simulink model "Model_2b_H2_batteries_secundary_clean"  (R2019a)
settings: Solver=FixedStepAuto  StartTime=0.0  StopTime=8760  FixedStep=1  RelTol=1e-3
libraries: simulink x8
settings Model: Creator=senja  LastModifiedBy=senja

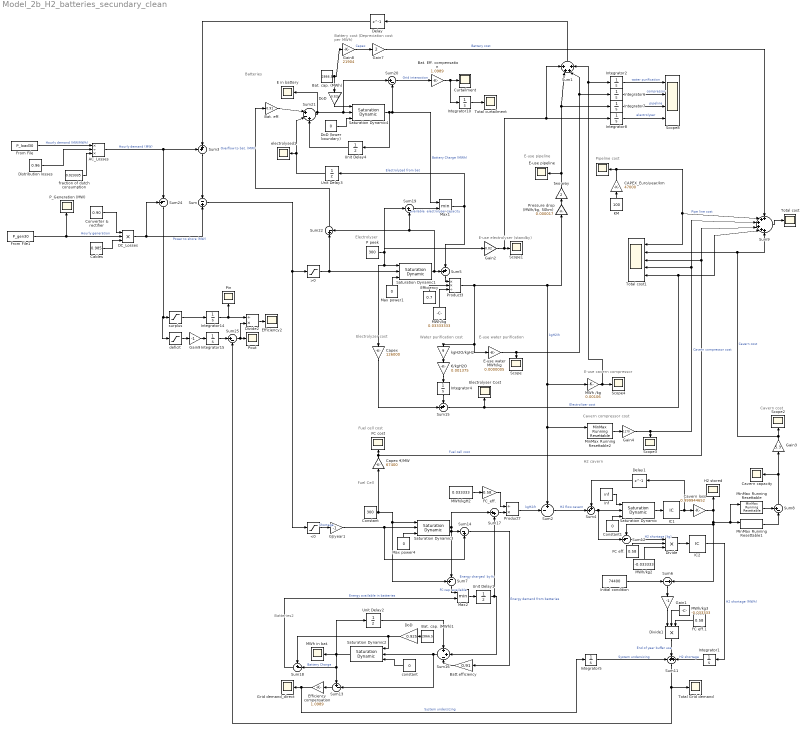
== system Model_2b_H2_batteries_secundary_clean ==
  note: Water purification cost
  note: E-use pipeline
  note: E-use cavern compressor
  note: Cavern compressor cost
  note: Cavern cost
  note: E-use electrolyser (standby)
  note: E-use water purification
  note: Fuel cell cost
  note: Pipeline cost
  note: H2 cavern
  note: Fuel Cell
  note: Electrolyser
  note: Electrolyzer cost
  note: Battery cost (Depreciation cost per MWh)
  note: Batteries
  note: Batteries2
  " " : Scope
  <0 : Saturate  UpperLimit=0  LowerLimit=-inf
  >0 : Saturate  UpperLimit=inf  LowerLimit=0
  AC_Losses : Product  Inputs=*/*
  "Bat. Eff. compensation " : Gain  Gain=1.0989
  Bat. cap. (MWh) : Constant  Value=2866.5
  Bat. cap. (MWh)1 : Constant  Value=2866.5
  Bat. eff. : Gain  Gain=0.91
  Batt.efficiency : Gain  Gain=0.91
  CAPEX_Euro/year/km : Gain  Gain=47000
  Cables : Constant  Value=0.985
  Capex : Gain  Gain=126000
  Capex €/MW : Gain  Gain=67400
  Cavern capacity : Scope
  Cavern loss : Gain  Gain=0.999944652
  Constant : Constant  Value=300
  Constant1 : Constant  Value=0
  Converter & rectifier : Constant  Value=0.90
  Curtailment : Scope
  DC_Losses : Product  Inputs=3
  Delay : Delay  DelayLength=1  InitialCondition=0
  Delay1 : Delay  DelayLength=1  InitialCondition=0
  Distribution losses : Constant  Value=0.96
  Divide : Product  Inputs=***
  Divide1 : Product  Inputs=***
  Divide2 : Product  Inputs=/*
  DoD : Gain  Gain=0.925
  "DoD " : Gain  Gain=0.925
  DoD (lower boundary) : Constant  Value=0
  E in battery : Scope
  E-use pipeline : Scope
  E-use water MWh/kg : Gain  Gain=0.0000005
  Efficiency : Constant  Value=0.7
  Efficiency compensation : Gain  Gain=1.0989
  Efficiency2 : Scope
  Electrolyser Cost : Scope
  FC cost : Scope
  FC eff. : Constant  Value=0.58
  FC eff.1 : Constant  Value=0.58
  FC_eff. : Gain  Gain=0.58
  From File : FromFile  FileName=P_load30  SampleTime=0
  From File1 : FromFile  FileName=P_gen30  SampleTime=0
  GJ/year1 : Gain  Gain=-1
  Gain1 : Gain  Gain=-1
  Gain2 : Gain  Gain=0.02
  Gain3 : Gain  Gain=5.3
  Gain4 : Gain  Gain=1170
  Gain7 : Gain  Gain=2
  Gain8 : Gain  Gain=21904
  Gain9 : Gain  Gain=-1
  Grid demand_direct : Scope
  "H2 stored " : Scope
  IC1 : InitialCondition  Value=74400
  IC2 : InitialCondition  Value=0
  Inf : Constant  Value=inf  OutDataTypeStr=Inherit: Inherit via back propagation
  Initial condition : Constant  Value=74400
  Integrator{1..2,4..8,10,14..15} (10 alike) : Integrator
  KM : Constant  Value=100
  MWh /kg : Gain  Gain=0.00106
  MWh in bat. : Scope
  MWh/kg : Constant  Value=0.03333333
  MWh/kg2 : Constant  Value=-0.033333
  MWh/kg3 : Constant  Value=-0.033333
  MWh/kgH2 : Constant  Value=0.033333
  Max power1 : Constant  Value=0
  Max power4 : Constant  Value=0
  Max1 : MinMax  Inputs=2
  Max2 : MinMax  Inputs=2
  MinMax Running Resettable : simulink/Math Operations/MinMax Running Resettable  Function=max  vinit=0.0
  MinMax Running Resettable1 : simulink/Math Operations/MinMax Running Resettable  Function=min  vinit=0.0
  MinMax Running Resettable2 : simulink/Math Operations/MinMax Running Resettable  Function=max  vinit=0.0
  P peek : Constant  Value=300
  P_Generation (MW) : Scope
  Pin : Scope
  Pout : Scope
  "Pressure drop (MWh/kg, 50km)" : Gain  Gain=0.000017
  Product3 : Product  Inputs=**/
  Product7 : Product  Inputs=/*
  Saturation Dynamic : simulink/Discontinuities/Saturation Dynamic  OutMin=0  OutMax=[]  OutDataTypeStr=Inherit: Same as second input  OutDataType=fixdt(1, 16)  OutScaling=2^-10  DoSatur=off
  Saturation Dynamic{1..4} (4 alike) : simulink/Discontinuities/Saturation Dynamic  OutMin=[]  OutMax=[]  OutDataTypeStr=Inherit: Same as second input  OutDataType=fixdt(1, 16)  OutScaling=2^-10  DoSatur=off
  Scope{,1..4} (5 alike) : Scope
  Scope8 : Scope  NumInputPorts=4
  Sum : Sum  Inputs=-|+
  Sum1 : Sum  Inputs=++++
  Sum11 : Sum  Inputs=+++
  Sum12 : Sum  Inputs=-+|
  Sum{2,7..8,13,18,24} (6 alike) : Sum  Inputs=+-|
  Sum14 : Sum  Inputs=|-+
  Sum{3..5,15} (4 alike) : Sum  Inputs=++|
  Sum16 : Sum  Inputs=++-
  Sum17 : Sum  Inputs=|++
  Sum{19..20,22,25} (4 alike) : Sum  Inputs=|+-
  Sum21 : Sum  Inputs=|+-+
  Sum6 : Sum  Inputs=-|+
  Sum9 : Sum  Inputs=++++++
  Total Grid demand : Scope
  Total cost : Scope
  Total cost1 : Scope  NumInputPorts=5
  Total curtailment : Scope
  Unit Delay{1..4} (4 alike) : UnitDelay  SampleTime=-1  HasFrameUpgradeWarning=on
  "constant " : Constant  Value=0
  deficit : Saturate  UpperLimit=0  LowerLimit=-inf
  electrolysed1 : Scope
  fraction of dutch consumption : Constant  Value=0.023335
  kgH2O/kgH2 : Gain  Gain=9
  surplus : Saturate  UpperLimit=inf  LowerLimit=0
  two-way : Gain  Gain=2
  €/kgH2O : Gain  Gain=0.001375
  wires:
  From File/1 -> AC_Losses/1  "Hourly demand (MW/MWh)"
  Efficiency/1 -> Product3/2
  fraction of dutch consumption/1 -> AC_Losses/3
  Distribution losses/1 -> AC_Losses/2
  Cables/1 -> DC_Losses/3
  Converter & rectifier/1 -> DC_Losses/1
  DC_Losses/1 -> Sum/2, Sum24/1  "Power to shore (MW)"
  <0/1 -> GJ/year1/1  "Shortage"
  AC_Losses/1 -> Sum3/1, Sum24/2  "Hourly demand (MW)"
  From File1/1 -> P_Generation (MW)/1, DC_Losses/2  "Hourly generation"
  Max power1/1 -> Saturation Dynamic1/3
  Capex/1 -> Sum15/2
  Sum15/1 -> Sum9/5, Total cost1/5, Electrolyser Cost/1  "Electrolizer cost"
  €/kgH2O/1 -> Integrator4/1
  GJ/year1/1 -> Saturation Dynamic3/2, Sum14/2
  KM/1 -> CAPEX_Euro/year/km/1
  CAPEX_Euro/year/km/1 -> Total cost1/1, Sum9/2, " "/1  "Pipe line cost"
  Product3/1 -> Sum2/1, MinMax Running Resettable2/1, MWh /kg/1, "Pressure drop (MWh/kg, 50km)"/1, E-use water MWh/kg/1, kgH2O/kgH2/1  "kgH2/h"
  Sum9/1 -> Total cost/1
  Constant/1 -> Sum7/1, Saturation Dynamic3/1, Capex €/MW/1
  Max power4/1 -> Saturation Dynamic3/3
  Saturation Dynamic3/1 -> Sum17/1, Sum7/2, Sum14/1
  MWh/kgH2/1 -> FC_eff./1
  kgH2O/kgH2/1 -> €/kgH2O/1
  Integrator4/1 -> Sum15/1
  MWh/kg/1 -> Product3/3
  Capex €/MW/1 -> Sum9/4, Total cost1/3, FC cost/1  "Fuel cell cost"
  FC_eff./1 -> Product7/1
  Product7/1 -> Sum2/2  "kgH2/h"
  MinMax Running Resettable/1 -> Sum8/1
  MinMax Running Resettable1/1 -> Sum8/2
  Sum8/1 -> Cavern capacity/1, Gain3/1
  FC eff./1 -> Divide/2
  MWh/kg2/1 -> Divide/3
  Divide/1 -> IC2/1
  Initial condition/1 -> Sum6/1
  Integrator5/1 -> Sum11/1  "System undersizing"
  Sum6/1 -> Gain1/1
  Gain1/1 -> Divide1/1
  E-use water MWh/kg/1 -> Sum1/3, Integrator6/1, Scope/1
  Gain2/1 -> Sum1/1, Integrator8/1, Scope1/1
  Gain3/1 -> Total cost1/2, Sum9/6, Scope2/1  "Cavern cost"
  MinMax Running Resettable2/1 -> Gain4/1
  Gain4/1 -> Scope3/1, Sum9/3, Total cost1/4  "Cavern compressor cost"
  MWh /kg/1 -> Scope4/1, Integrator2/1, Sum1/4
  "Pressure drop (MWh/kg, 50km)"/1 -> two-way/1
  two-way/1 -> E-use pipeline/1, Integrator7/1, Sum1/2
  Sum3/1 -> Sum/1
  Sum1/1 -> Delay/1
  Delay/1 -> Sum3/2
  MWh/kg3/1 -> Divide1/2
  FC eff.1/1 -> Divide1/3
  Divide1/1 -> Sum11/2  "End of year buffer use"
  Cavern loss/1 -> Sum6/2, Sum12/1, MinMax Running Resettable1/1, MinMax Running Resettable/1, "H2 stored "/1
  Sum12/1 -> Divide/1  "H2 shortage (kg)"
  Delay1/1 -> Sum4/1
  Constant1/1 -> Saturation Dynamic/3
  Saturation Dynamic/1 -> IC1/1
  Sum4/1 -> Sum12/2, Saturation Dynamic/2
  IC1/1 -> Delay1/1, Cavern loss/1
  Sum2/1 -> Sum4/2  "H2 flow cavern"
  Inf/1 -> Saturation Dynamic/1
  IC2/1 -> Integrator1/1  "H2 shortage (MWh)"
  Integrator2/1 -> Scope8/1  "water purification"
  Integrator6/1 -> Scope8/2  "compressor"
  Integrator7/1 -> Scope8/3  "pipeline"
  Integrator8/1 -> Scope8/4  "electrolyser"
  Max1/1 -> Unit Delay3/1, Sum5/2  "Electrolyzed from bat"
  Bat. eff./1 -> Sum21/1
  Unit Delay4/1 -> Sum21/3
  Sum22/1 -> Bat. eff./1  "Overflow to bat. (MW)"
  DoD (lower boundary)/1 -> Saturation Dynamic4/3
  Sum21/1 -> Saturation Dynamic4/2, Sum20/1, E in battery/1
  Integrator10/1 -> Total curtailment/1
  Sum19/1 -> Max1/2  "available  electrolyser capacity"
  Unit Delay3/1 -> electrolysed1/1, Sum21/2
  Saturation Dynamic1/1 -> Sum5/1, Sum22/2, Sum19/2
  Gain8/1 -> Gain7/1  "Capex"
  Sum20/1 -> "Bat. Eff. compensation "/1  "Grid interaction"
  Saturation Dynamic4/1 -> Max1/1, Sum20/2, Unit Delay4/1  "Battery Charge (MWh)"
  >0/1 -> Saturation Dynamic1/2, Sum22/1
  Bat. cap. (MWh)/1 -> Gain8/1, "DoD "/1
  P peek/1 -> Gain2/1, Capex/1, Saturation Dynamic1/1, Sum19/1
  Sum5/1 -> Product3/1
  "DoD "/1 -> Saturation Dynamic4/1
  Bat. cap. (MWh)1/1 -> DoD/1
  Saturation Dynamic2/1 -> Sum18/2, Sum13/1, Unit Delay2/1, MWh in bat./1  "Battery Charge"
  DoD/1 -> Sum18/1, Saturation Dynamic2/1
  Sum13/1 -> Efficiency compensation/1
  Sum18/1 -> Max2/2  "Energy available in batteries"
  Batt.efficiency/1 -> Sum16/3
  "constant "/1 -> Saturation Dynamic2/3
  Sum16/1 -> Sum13/2, Saturation Dynamic2/2
  Unit Delay1/1 -> Sum16/2, Sum17/2  "Energy charged  by fc"
  Unit Delay2/1 -> Sum16/1
  Max2/1 -> Unit Delay1/1
  Sum14/1 -> Batt.efficiency/1  "Energy demand from batteries"
  Sum7/1 -> Max2/1  "FC cap. available"
  Gain7/1 -> Sum9/1  "Battery cost"
  Efficiency compensation/1 -> Integrator5/1, Grid demand_direct/1  "System undersizing"
  "Bat. Eff. compensation "/1 -> Curtailment/1, Integrator10/1
  Sum17/1 -> Product7/2
  Sum11/1 -> Sum25/2, Total Grid demand/1
  deficit/1 -> Gain9/1
  Sum24/1 -> deficit/1, surplus/1
  Gain9/1 -> Integrator15/1
  Sum25/1 -> Divide2/2, Pout/1
  Integrator14/1 -> Divide2/1, Pin/1
  surplus/1 -> Integrator14/1
  Integrator15/1 -> Sum25/1
  Sum/1 -> <0/1, >0/1
  Integrator1/1 -> Sum11/3  "H2 shortage"
  Divide2/1 -> Efficiency2/1
